simulink library "ammclib_bam"  (Simulink 9.3)
(part 5 of 21)

      |         add_block('built-in/Inport', [gcb, '/s16IntegGainShiftQ'], 'Position', pos, 'Orientation', orient, 'OutDataTypeStr', 'int16');
      | 
      |         pos = get_param(    [gcb, '/f32LowerLimitQ'], 'Position');
      |         orient = get_param( [gcb, '/f32LowerLimitQ'], 'Orientation');
      |         delete_block(       [gcb, '/f32LowerLimitQ']);
      |         add_block('built-in/Inport', [gcb, '/f32LowerLimitQ'], 'Position', pos, 'Orientation', orient, 'OutDataTypeStr', 'int32');
      | 
      |         pos = get_param(    [gcb, '/f32UpperLimitQ'], 'Position');
      |         orient = get_param( [gcb, '/f32UpperLimitQ'], 'Orientation');
      |         delete_block(       [gcb, '/f32UpperLimitQ']);
      |         add_block('built-in/Inport', [gcb, '/f32UpperLimitQ'], 'Position', pos, 'Orientation', orient, 'OutDataTypeStr', 'int32');
      | 
      |         pos = get_param(    [gcb, '/f32RampUp'], 'Position');
      |         orient = get_param( [gcb, '/f32RampUp'], 'Orientation');
      |         delete_block(       [gcb, '/f32RampUp']);
      |         add_block('built-in/Inport', [gcb, '/f32RampUp'], 'Position', pos, 'Orientation', orient, 'OutDataTypeStr', 'int32');
      | 
      |         pos = get_param(    [gcb, '/f32RampDown'], 'Position');
      |         orient = get_param( [gcb, '/f32RampDown'], 'Orientation');
      |         delete_block(       [gcb, '/f32RampDown']);
      |         add_block('built-in/Inport', [gcb, '/f32RampDown'], 'Position', pos, 'Orientation', orient, 'OutDataTypeStr', 'int32');
      | 
      |         pos = get_param(    [gcb, '/f32AccW'], 'Position');
      |         orient = get_param( [gcb, '/f32AccW'], 'Orientation');
      |         delete_block(       [gcb, '/f32AccW']);
      |         add_block('built-in/Inport', [gcb, '/f32AccW'], 'Position', pos, 'Orientation', orient, 'OutDataTypeStr', 'int32');
      | 
      |         pos = get_param(    [gcb, '/f32IntegPartK_1Q'], 'Position');
      |         orient = get_param( [gcb, '/f32IntegPartK_1Q'], 'Orientation');
      |         delete_block(       [gcb, '/f32IntegPartK_1Q']);
      |         add_block('built-in/Inport', [gcb, '/f32IntegPartK_1Q'], 'Position', pos, 'Orientation', orient, 'OutDataTypeStr', 'int32');
      | 
      |         pos = get_param(    [gcb, '/f32InK_1Q'], 'Position');
      |         orient = get_param( [gcb, '/f32InK_1Q'], 'Orientation');
      |         delete_block(       [gcb, '/f32InK_1Q']);
      |         add_block('built-in/Inport', [gcb, '/f32InK_1Q'], 'Position', pos, 'Orientation', orient, 'OutDataTypeStr', 'int32');
      | 
      |         pos = get_param(    [gcb, '/f32State'], 'Position');
      |         orient = get_param( [gcb, '/f32State'], 'Orientation');
      |         delete_block(       [gcb, '/f32State']);
      |         add_block('built-in/Inport', [gcb, '/f32State'], 'Position', pos, 'Orientation', orient, 'OutDataTypeStr', 'int32');
      | 
      | 
      |         pos = get_param(    [gcb '/f32AccW_Out'], 'Position');
      |         orient = get_param( [gcb '/f32AccW_Out'], 'Orientation');
      |         delete_block(       [gcb '/f32AccW_Out']);
      |         add_block('built-in/Outport', [gcb '/f32AccW_Out'], 'Position', pos, 'Orientation', orient);
      | 
      |         pos = get_param(    [gcb '/f32IntegPartK_1Q_Out'], 'Position');
      |         orient = get_param( [gcb '/f32IntegPartK_1Q_Out'], 'Orientation');
      |         delete_block(       [gcb '/f32IntegPartK_1Q_Out']);
      |         add_block('built-in/Outport', [gcb '/f32IntegPartK_1Q_Out'], 'Position', pos, 'Orientation', orient);
      | 
      |         pos = get_param(    [gcb '/f32InK_1Q_Out'], 'Position');
      |         orient = get_param( [gcb '/f32InK_1Q_Out'], 'Orientation');
      |         delete_block(       [gcb '/f32InK_1Q_Out']);
      |         add_block('built-in/Outport', [gcb '/f32InK_1Q_Out'], 'Position', pos, 'Orientation', orient);
      | 
      |         pos = get_param(    [gcb '/f32State_Out'], 'Position');
      |         orient = get_param( [gcb '/f32State_Out'], 'Orientation');
      |         delete_block(       [gcb '/f32State_Out']);
      |         add_block('built-in/Outport', [gcb '/f32State_Out'], 'Position', pos, 'Orientation', orient);
      | 
      | 
      |         if (showDebugOutputs == 2) && (strcmp(get_param([gcb '/f32WReqFilt'], 'BlockType'), 'Terminator'))
      |             pos = get_param(    [gcb '/f32WReqFilt'], 'Position');
      |             orient = get_param( [gcb '/f32WReqFilt'], 'Orientation');
      |             delete_block(       [gcb '/f32WReqFilt']);
      |             add_block('built-in/Outport', [gcb '/f32WReqFilt'], 'Position', pos, 'Orientation', orient);
      | 
      |             pos = get_param(    [gcb '/f32WErr'], 'Position');
      |             orient = get_param( [gcb '/f32WErr'], 'Orientation');
      |             delete_block(       [gcb '/f32WErr']);
      |             add_block('built-in/Outport', [gcb '/f32WErr'], 'Position', pos, 'Orientation', orient);
      | 
      |             pos = get_param(    [gcb '/f32WFbckFilt'], 'Position');
      |             orient = get_param( [gcb '/f32WFbckFilt'], 'Orientation');
      |             delete_block(       [gcb '/f32WFbckFilt']);
      |             add_block('built-in/Outport', [gcb '/f32WFbckFilt'], 'Position', pos, 'Orientation', orient);
      | 
      |         end
      | 
      |         set_param([gcb '/f32VelocityReq'], 'Port', '1');
      |         set_param([gcb '/f32VelocityFbck'], 'Port', '2');
      |         set_param([gcb '/f32FilterMAWOut_preset'], 'Port', '3');
      |         set_param([gcb '/f32ControllerPIpAWQOut_preset'], 'Port', '4');
      |         set_param([gcb '/f32RampOut_preset'], 'Port', '5');
      |         set_param([gcb '/u16NSamplesW'], 'Port', '6');
      |         set_param([gcb '/f32PropGainQ'], 'Port', '7');
      |         set_param([gcb '/f32IntegGainQ'], 'Port', '8');
      |         set_param([gcb '/s16PropGainShiftQ'], 'Port', '9');
      |         set_param([gcb '/s16IntegGainShiftQ'], 'Port', '10');
      |         set_param([gcb '/f32LowerLimitQ'], 'Port', '11');
      |         set_param([gcb '/f32UpperLimitQ'], 'Port', '12');
      |         set_param([gcb '/f32RampUp'], 'Port', '13');
      |         set_param([gcb '/f32RampDown'], 'Port', '14');
      |         set_param([gcb '/f32AccW'], 'Port', '15');
      |         set_param([gcb '/f32IntegPartK_1Q'], 'Port', '16');
      |         set_param([gcb '/f32InK_1Q'], 'Port', '17');
      |         set_param([gcb '/f32State'], 'Port', '18');
      | 
      |         if (showDebugOutputs == 2)
      |             set_param([gcb '/pIDQReq'], 'Port', '1');
      |             set_param([gcb '/u16LimitFlagQ'], 'Port', '2');
      |             set_param([gcb '/f32WReqFilt'], 'Port', '3');
      |             set_param([gcb '/f32WErr'], 'Port', '4');
      |             set_param([gcb '/f32WFbckFilt'], 'Port', '5');
      |             set_param([gcb '/f32AccW_Out'], 'Port', '6');
      |             set_param([gcb '/f32IntegPartK_1Q_Out'], 'Port', '7');
      |             set_param([gcb '/f32InK_1Q_Out'], 'Port', '8');
      |             set_param([gcb '/f32State_Out'], 'Port', '9');
      |         else
      |             set_param([gcb '/pIDQReq'], 'Port', '1');
      |             set_param([gcb '/u16LimitFlagQ'], 'Port', '2');
      |             set_param([gcb '/f32AccW_Out'], 'Port', '3');
      |             set_param([gcb '/f32IntegPartK_1Q_Out'], 'Port', '4');
      |             set_param([gcb '/f32InK_1Q_Out'], 'Port', '5');
      |             set_param([gcb '/f32State_Out'], 'Port', '6');
      |         end
      | 
      |         set_param(gcb,'MaskEnables',{'on','on','on','off','off','off','off','off','off','off','off','off'});
      | 
      |         if (posblk(4) - posblk(2)) < 475
      |           height = 475;
      |           set_param(gcb,'Position',[posblk(1), posblk(2), posblk(3), posblk(2)+height])
      |         end
      |     else
      |         if (showDebugOutputs == 2) && (strcmp(get_param([gcb '/f32WReqFilt'], 'BlockType'), 'Terminator'))
      |             % shown debugging outputs
      |             pos = get_param(    [gcb '/f32WReqFilt'], 'Position');
      |             orient = get_param( [gcb '/f32WReqFilt'], 'Orientation');
      |             delete_block(       [gcb '/f32WReqFilt']);
      |             add_block('built-in/Outport', [gcb '/f32WReqFilt'], 'Position', pos, 'Orientation', orient);
      | 
      |             pos = get_param(    [gcb '/f32WErr'], 'Position');
      |             orient = get_param( [gcb '/f32WErr'], 'Orientation');
      |             delete_block(       [gcb '/f32WErr']);
      |             add_block('built-in/Outport', [gcb '/f32WErr'], 'Position', pos, 'Orientation', orient);
      | 
      |             pos = get_param(    [gcb '/f32WFbckFilt'], 'Position');
      |             orient = get_param( [gcb '/f32WFbckFilt'], 'Orientation');
      |             delete_block(       [gcb '/f32WFbckFilt']);
      |             add_block('built-in/Outport', [gcb '/f32WFbckFilt'], 'Position', pos, 'Orientation', orient);
      | 
      |             set_param([gcb '/pIDQReq'], 'Port', '1');
      |             set_param([gcb '/u16LimitFlagQ'], 'Port', '2');
      |             set_param([gcb '/f32WReqFilt'], 'Port', '3');
      |             set_param([gcb '/f32WErr'], 'Port', '4');
      |             set_param([gcb '/f32WFbckFilt'], 'Port', '5');
      |             set_param([gcb '/f32AccW_Out'], 'Port', '6');
      |             set_param([gcb '/f32IntegPartK_1Q_Out'], 'Port', '7');
      |             set_param([gcb '/f32InK_1Q_Out'], 'Port', '8');
      |             set_param([gcb '/f32State_Out'], 'Port', '9');
      |         elseif (showDebugOutputs == 1) && (strcmp(get_param([gcb '/f32WReqFilt'], 'BlockType'), 'Outport'))
      |             % hidden debugging outputs
      |             pos = get_param(    [gcb '/f32WReqFilt'], 'Position');
      |             orient = get_param( [gcb '/f32WReqFilt'], 'Orientation');
      |             delete_block(       [gcb '/f32WReqFilt']);
      |             add_block('built-in/Terminator', [gcb '/f32WReqFilt'], 'Position', pos, 'Orientation', orient);
      | 
      |             pos = get_param(    [gcb '/f32WErr'], 'Position');
      |             orient = get_param( [gcb '/f32WErr'], 'Orientation');
      |             delete_block(       [gcb '/f32WErr']);
      |             add_block('built-in/Terminator', [gcb '/f32WErr'], 'Position', pos, 'Orientation', orient);
      | 
      |             pos = get_param(    [gcb '/f32WFbckFilt'], 'Position');
      |             orient = get_param( [gcb '/f32WFbckFilt'], 'Orientation');
      |             delete_block(       [gcb '/f32WFbckFilt']);
      |             add_block('built-in/Terminator', [gcb '/f32WFbckFilt'], 'Position', pos, 'Orientation', orient);
      | 
      |             set_param([gcb '/pIDQReq'], 'Port', '1');
      |             set_param([gcb '/u16LimitFlagQ'], 'Port', '2');
      |             set_param([gcb '/f32AccW_Out'], 'Port', '3');
      |             set_param([gcb '/f32IntegPartK_1Q_Out'], 'Port', '4');
      |             set_param([gcb '/f32InK_1Q_Out'], 'Port', '5');
      |             set_param([gcb '/f32State_Out'], 'Port', '6');
      |         end
      |     end
      | end
      settings: RTWSystemCode=Inline
      mask TypeOptions showStates: Hide (faster execution) | Show (allows debugging; connect feedback loops manually)
      mask Callback showStates:
      | maskStr = get_param(gcb,'showStates');
      | if strcmp(maskStr,'Hide (faster execution)'),
      |     set_param(gcb,'MaskEnables',{'on','on','off','on','on','on','on','on','on','on','on','on'});
      | else
      |     set_param(gcb,'MaskEnables',{'on','on','on','off','off','off','off','off','off','off','off','off'});
      | end
      mask TypeOptions resetStatesEnable: Pre-set according to the first set of inputs after reset | Clear to zero
      mask TypeOptions showDebugOutputs: Hide | Show
      mask Display:
      | color('black');
      | pos = get_param(gcb, 'Position');
      | width = pos(3) - pos(1);
      | height = pos(4) - pos(2);
      | tX=width/2;
      | tY=height - 25;
      | color('black');
      | text(tX,tY, 'AMCLIB_SpeedLoop_F32', 'horizontalAlignment', 'center');
      | if showStates == 2
      |   color('red');
      |   text(tX,tY - 20, ['debugging mode' char(13) char(10) '(limited performance)'], 'horizontalAlignment', 'center');
      | end
  AMCLIB_TrackObsrv_F32 : Subsystem  TreatAsAtomicUnit=on  mask(AMCLIB_TrackObsrv_F32){showStates=Hide (faster execution), resetStatesEnable=Pre-set according to the first set of inputs after reset, f32CC1sc=0, f32CC2sc=0, f32UpperLimit=0, f32LowerLimit=0, u16NShiftPI=0, f32C1=0, u16NShiftI=0}
      mask prompts: showStates "Show internal states"; resetStatesEnable "Internal state after reset"; f32CC1sc "f32CC1sc (GFLIB_ControllerPIrAW - CC1 coefficient)"; f32CC2sc "f32CC2sc (GFLIB_ControllerPIrAW - CC2 coefficient)"; f32UpperLimit "f32UpperLimit (GFLIB_ControllerPIrAW - upper Limit of the controller)"; f32LowerLimit "f32LowerLimit (GFLIB_ControllerPIrAW - lower Limit of the controller)"; u16NShiftPI "u16NShiftPI (GFLIB_ControllerPIrAW - scaling bitwise shift applied to the controller coefficients)"; f32C1 "f32C1 (GFLIB_IntegratorTR - integrator coefficient)"; u16NShiftI "u16NShiftI (GFLIB_IntegratorTR - scaling bitwise shift applied to the integrator coefficient)"
      mask help: Tracking observer in 32-bit fixed-point fractional implementation. This block supports re-initialization of the internal state during simulation. If the block is reset, the outputs of the PI controller and integrator will be aligned with the inputs f32VelocityOut_preset and f32PosOut_preset. Refer to the AMMCLIB User's Guide for further details.
      mask init:
      | if ~evalin('base','exist(''tS8'',''var'')')
      |   if (2 ~= exist('SWLIBS_Typedefs.mat','file'))
      |       error('File SWLIBS_Typedefs.mat is not on the Matlab path. Please add the AMMCLIB "bam" folder in the Matlab Search Path.');
      |   else
      |       evalin('base', 'load(''SWLIBS_Typedefs.mat'')');
      |   end
      | end
      | if showStates == 1
      |     % hidden state variables
      |     if strcmp(get_param([gcb '/f32CC1sc'], 'BlockType'), 'Inport')
      |         posblk = get_param(gcb, 'Position');
      | 
      |         pos = get_param(    [gcb, '/f32CC1sc'], 'Position');
      |         orient = get_param( [gcb, '/f32CC1sc'], 'Orientation');
      |         delete_block(       [gcb, '/f32CC1sc']);
      |         add_block('built-in/Ground', [gcb, '/f32CC1sc'], 'Position', pos, 'Orientation', orient);
      | 
      |         pos = get_param(    [gcb, '/f32CC2sc'], 'Position');
      |         orient = get_param( [gcb, '/f32CC2sc'], 'Orientation');
      |         delete_block(       [gcb, '/f32CC2sc']);
      |         add_block('built-in/Ground', [gcb, '/f32CC2sc'], 'Position', pos, 'Orientation', orient);
      | 
      |         pos = get_param(    [gcb, '/f32UpperLimit'], 'Position');
      |         orient = get_param( [gcb, '/f32UpperLimit'], 'Orientation');
      |         delete_block(       [gcb, '/f32UpperLimit']);
      |         add_block('built-in/Ground', [gcb, '/f32UpperLimit'], 'Position', pos, 'Orientation', orient);
      | 
      |         pos = get_param(    [gcb, '/f32LowerLimit'], 'Position');
      |         orient = get_param( [gcb, '/f32LowerLimit'], 'Orientation');
      |         delete_block(       [gcb, '/f32LowerLimit']);
      |         add_block('built-in/Ground', [gcb, '/f32LowerLimit'], 'Position', pos, 'Orientation', orient);
      | 
      |         pos = get_param(    [gcb, '/u16NShiftPI'], 'Position');
      |         orient = get_param( [gcb, '/u16NShiftPI'], 'Orientation');
      |         delete_block(       [gcb, '/u16NShiftPI']);
      |         add_block('built-in/Ground', [gcb, '/u16NShiftPI'], 'Position', pos, 'Orientation', orient);
      | 
      |         pos = get_param(    [gcb, '/f32C1'], 'Position');
      |         orient = get_param( [gcb, '/f32C1'], 'Orientation');
      |         delete_block(       [gcb, '/f32C1']);
      |         add_block('built-in/Ground', [gcb, '/f32C1'], 'Position', pos, 'Orientation', orient);
      | 
      |         pos = get_param(    [gcb, '/u16NShiftI'], 'Position');
      |         orient = get_param( [gcb, '/u16NShiftI'], 'Orientation');
      |         delete_block(       [gcb, '/u16NShiftI']);
      |         add_block('built-in/Ground', [gcb, '/u16NShiftI'], 'Position', pos, 'Orientation', orient);
      | 
      |         pos = get_param(    [gcb, '/f32Acc'], 'Position');
      |         orient = get_param( [gcb, '/f32Acc'], 'Orientation');
      |         delete_block(       [gcb, '/f32Acc']);
      |         add_block('built-in/Ground', [gcb, '/f32Acc'], 'Position', pos, 'Orientation', orient);
      | 
      |         pos = get_param(    [gcb, '/f32InErrK1'], 'Position');
      |         orient = get_param( [gcb, '/f32InErrK1'], 'Orientation');
      |         delete_block(       [gcb, '/f32InErrK1']);
      |         add_block('built-in/Ground', [gcb, '/f32InErrK1'], 'Position', pos, 'Orientation', orient);
      | 
      |         pos = get_param(    [gcb, '/f32State'], 'Position');
      |         orient = get_param( [gcb, '/f32State'], 'Orientation');
      |         delete_block(       [gcb, '/f32State']);
      |         add_block('built-in/Ground', [gcb, '/f32State'], 'Position', pos, 'Orientation', orient);
      | 
      |         pos = get_param(    [gcb, '/f32InK1'], 'Position');
      |         orient = get_param( [gcb, '/f32InK1'], 'Orientation');
      |         delete_block(       [gcb, '/f32InK1']);
      |         add_block('built-in/Ground', [gcb, '/f32InK1'], 'Position', pos, 'Orientation', orient);
      | 
      | 
      |         pos = get_param(    [gcb '/f32Acc_Out'], 'Position');
      |         orient = get_param( [gcb '/f32Acc_Out'], 'Orientation');
      |         delete_block(       [gcb '/f32Acc_Out']);
      |         add_block('built-in/Terminator', [gcb '/f32Acc_Out'], 'Position', pos, 'Orientation', orient);
      | 
      |         pos = get_param(    [gcb '/f32InErrK1_Out'], 'Position');
      |         orient = get_param( [gcb '/f32InErrK1_Out'], 'Orientation');
      |         delete_block(       [gcb '/f32InErrK1_Out']);
      |         add_block('built-in/Terminator', [gcb '/f32InErrK1_Out'], 'Position', pos, 'Orientation', orient);
      | 
      |         pos = get_param(    [gcb '/f32State_Out'], 'Position');
      |         orient = get_param( [gcb '/f32State_Out'], 'Orientation');
      |         delete_block(       [gcb '/f32State_Out']);
      |         add_block('built-in/Terminator', [gcb '/f32State_Out'], 'Position', pos, 'Orientation', orient);
      | 
      |         pos = get_param(    [gcb '/f32InK1_Out'], 'Position');
      |         orient = get_param( [gcb '/f32InK1_Out'], 'Orientation');
      |         delete_block(       [gcb '/f32InK1_Out']);
      |         add_block('built-in/Terminator', [gcb '/f32InK1_Out'], 'Position', pos, 'Orientation', orient);
      | 
      | 
      |         set_param([gcb '/f32PhaseErr'], 'Port', '1');
      |         set_param([gcb '/f32VelocityOut_preset'], 'Port', '2');
      |         set_param([gcb '/f32PosOut_preset'], 'Port', '3');
      | 
      |         set_param([gcb '/pPosEst'], 'Port', '1');
      |         set_param([gcb '/pVelocityEst'], 'Port', '2');
      | 
      |         set_param(gcb,'MaskEnables',{'on','on','on','on','on','on','on','on','on'});
      | 
      |         if (posblk(4) - posblk(2)) > 100
      |           height = 100;
      |           set_param(gcb,'Position',[posblk(1), posblk(2), posblk(3), posblk(2)+height])
      |         end
      |     end
      | else
      |     % shown state variables
      |     if strcmp(get_param([gcb '/f32CC1sc'], 'BlockType'), 'Ground')
      |         posblk = get_param(gcb, 'Position');
      | 
      |         pos = get_param(    [gcb, '/f32CC1sc'], 'Position');
      |         orient = get_param( [gcb, '/f32CC1sc'], 'Orientation');
      |         delete_block(       [gcb, '/f32CC1sc']);
      |         add_block('built-in/Inport', [gcb, '/f32CC1sc'], 'Position', pos, 'Orientation', orient, 'OutDataTypeStr', 'int32');
      | 
      |         pos = get_param(    [gcb, '/f32CC2sc'], 'Position');
      |         orient = get_param( [gcb, '/f32CC2sc'], 'Orientation');
      |         delete_block(       [gcb, '/f32CC2sc']);
      |         add_block('built-in/Inport', [gcb, '/f32CC2sc'], 'Position', pos, 'Orientation', orient, 'OutDataTypeStr', 'int32');
      | 
      |         pos = get_param(    [gcb, '/f32UpperLimit'], 'Position');
      |         orient = get_param( [gcb, '/f32UpperLimit'], 'Orientation');
      |         delete_block(       [gcb, '/f32UpperLimit']);
      |         add_block('built-in/Inport', [gcb, '/f32UpperLimit'], 'Position', pos, 'Orientation', orient, 'OutDataTypeStr', 'int32');
      | 
      |         pos = get_param(    [gcb, '/f32LowerLimit'], 'Position');
      |         orient = get_param( [gcb, '/f32LowerLimit'], 'Orientation');
      |         delete_block(       [gcb, '/f32LowerLimit']);
      |         add_block('built-in/Inport', [gcb, '/f32LowerLimit'], 'Position', pos, 'Orientation', orient, 'OutDataTypeStr', 'int32');
      | 
      |         pos = get_param(    [gcb, '/u16NShiftPI'], 'Position');
      |         orient = get_param( [gcb, '/u16NShiftPI'], 'Orientation');
      |         delete_block(       [gcb, '/u16NShiftPI']);
      |         add_block('built-in/Inport', [gcb, '/u16NShiftPI'], 'Position', pos, 'Orientation', orient, 'OutDataTypeStr', 'uint16');
      | 
      |         pos = get_param(    [gcb, '/f32C1'], 'Position');
      |         orient = get_param( [gcb, '/f32C1'], 'Orientation');
      |         delete_block(       [gcb, '/f32C1']);
      |         add_block('built-in/Inport', [gcb, '/f32C1'], 'Position', pos, 'Orientation', orient, 'OutDataTypeStr', 'int32');
      | 
      |         pos = get_param(    [gcb, '/u16NShiftI'], 'Position');
      |         orient = get_param( [gcb, '/u16NShiftI'], 'Orientation');
      |         delete_block(       [gcb, '/u16NShiftI']);
      |         add_block('built-in/Inport', [gcb, '/u16NShiftI'], 'Position', pos, 'Orientation', orient, 'OutDataTypeStr', 'uint16');
      | 
      |         pos = get_param(    [gcb, '/f32Acc'], 'Position');
      |         orient = get_param( [gcb, '/f32Acc'], 'Orientation');
      |         delete_block(       [gcb, '/f32Acc']);
      |         add_block('built-in/Inport', [gcb, '/f32Acc'], 'Position', pos, 'Orientation', orient, 'OutDataTypeStr', 'int32');
      | 
      |         pos = get_param(    [gcb, '/f32InErrK1'], 'Position');
      |         orient = get_param( [gcb, '/f32InErrK1'], 'Orientation');
      |         delete_block(       [gcb, '/f32InErrK1']);
      |         add_block('built-in/Inport', [gcb, '/f32InErrK1'], 'Position', pos, 'Orientation', orient, 'OutDataTypeStr', 'int32');
      | 
      |         pos = get_param(    [gcb, '/f32State'], 'Position');
      |         orient = get_param( [gcb, '/f32State'], 'Orientation');
      |         delete_block(       [gcb, '/f32State']);
      |         add_block('built-in/Inport', [gcb, '/f32State'], 'Position', pos, 'Orientation', orient, 'OutDataTypeStr', 'int32');
      | 
      |         pos = get_param(    [gcb, '/f32InK1'], 'Position');
      |         orient = get_param( [gcb, '/f32InK1'], 'Orientation');
      |         delete_block(       [gcb, '/f32InK1']);
      |         add_block('built-in/Inport', [gcb, '/f32InK1'], 'Position', pos, 'Orientation', orient, 'OutDataTypeStr', 'int32');
      | 
      | 
      |         pos = get_param(    [gcb '/f32Acc_Out'], 'Position');
      |         orient = get_param( [gcb '/f32Acc_Out'], 'Orientation');
      |         delete_block(       [gcb '/f32Acc_Out']);
      |         add_block('built-in/Outport', [gcb '/f32Acc_Out'], 'Position', pos, 'Orientation', orient);
      | 
      |         pos = get_param(    [gcb '/f32InErrK1_Out'], 'Position');
      |         orient = get_param( [gcb '/f32InErrK1_Out'], 'Orientation');
      |         delete_block(       [gcb '/f32InErrK1_Out']);
      |         add_block('built-in/Outport', [gcb '/f32InErrK1_Out'], 'Position', pos, 'Orientation', orient);
      | 
      |         pos = get_param(    [gcb '/f32State_Out'], 'Position');
      |         orient = get_param( [gcb '/f32State_Out'], 'Orientation');
      |         delete_block(       [gcb '/f32State_Out']);
      |         add_block('built-in/Outport', [gcb '/f32State_Out'], 'Position', pos, 'Orientation', orient);
      | 
      |         pos = get_param(    [gcb '/f32InK1_Out'], 'Position');
      |         orient = get_param( [gcb '/f32InK1_Out'], 'Orientation');
      |         delete_block(       [gcb '/f32InK1_Out']);
      |         add_block('built-in/Outport', [gcb '/f32InK1_Out'], 'Position', pos, 'Orientation', orient);
      | 
      | 
      |         set_param([gcb '/f32PhaseErr'], 'Port', '1');
      |         set_param([gcb '/f32VelocityOut_preset'], 'Port', '2');
      |         set_param([gcb '/f32PosOut_preset'], 'Port', '3');
      |         set_param([gcb '/f32CC1sc'], 'Port', '4');
      |         set_param([gcb '/f32CC2sc'], 'Port', '5');
      |         set_param([gcb '/f32UpperLimit'], 'Port', '6');
      |         set_param([gcb '/f32LowerLimit'], 'Port', '7');
      |         set_param([gcb '/u16NShiftPI'], 'Port', '8');
      |         set_param([gcb '/f32C1'], 'Port', '9');
      |         set_param([gcb '/u16NShiftI'], 'Port', '10');
      |         set_param([gcb '/f32Acc'], 'Port', '11');
      |         set_param([gcb '/f32InErrK1'], 'Port', '12');
      |         set_param([gcb '/f32State'], 'Port', '13');
      |         set_param([gcb '/f32InK1'], 'Port', '14');
      | 
      |         set_param([gcb '/pPosEst'], 'Port', '1');
      |         set_param([gcb '/pVelocityEst'], 'Port', '2');
      |         set_param([gcb '/f32Acc_Out'], 'Port', '3');
      |         set_param([gcb '/f32InErrK1_Out'], 'Port', '4');
      |         set_param([gcb '/f32State_Out'], 'Port', '5');
      |         set_param([gcb '/f32InK1_Out'], 'Port', '6');
      | 
      |         set_param(gcb,'MaskEnables',{'on','on','off','off','off','off','off','off','off'});
      | 
      |         if (posblk(4) - posblk(2)) < 375
      |           height = 375;
      |           set_param(gcb,'Position',[posblk(1), posblk(2), posblk(3), posblk(2)+height])
      |         end
      |     end
      | end
      settings: RTWSystemCode=Inline
      mask TypeOptions showStates: Hide (faster execution) | Show (allows debugging; connect feedback loops manually)
      mask Callback showStates:
      | maskStr = get_param(gcb,'showStates');
      | if strcmp(maskStr,'Hide (faster execution)'),
      |     set_param(gcb,'MaskEnables',{'on','on','on','on','on','on','on','on','on'});
      | else
      |     set_param(gcb,'MaskEnables',{'on','on','off','off','off','off','off','off','off'});
      | end
      mask TypeOptions resetStatesEnable: Pre-set according to the first set of inputs after reset | Clear to zero
      mask Display:
      | color('black');
      | pos = get_param(gcb, 'Position');
      | width = pos(3) - pos(1);
      | height = pos(4) - pos(2);
      | tX=width/2;
      | tY=height - 25;
      | color('black');
      | text(tX,tY, 'AMCLIB_TrackObsrv_F32', 'horizontalAlignment', 'center');
      | if showStates == 2
      |   color('red');
      |   text(tX,tY - 20, ['debugging mode' char(13) char(10) '(limited performance)'], 'horizontalAlignment', 'center');
      | end
  AMCLIB_Windmilling_F32 : Subsystem  TreatAsAtomicUnit=on  mask(AMCLIB_Windmilling_F32){showStates=Hide (faster execution), f32ADCMaxError=0, f32CC1sc=0, f32CC2sc=0, f32UpperLimit=0, f32LowerLimit=0, u16NShiftPI=0, f32C1=0, u16NShiftI=0}
      mask prompts: showStates "Show internal states"; f32ADCMaxError "f32ADCMaxError (Maximum differential offset error between any two phases of the 3-phase voltage-sensing A/D converters.)"; f32CC1sc "f32CC1sc (GFLIB_ControllerPIrAW - CC1 coefficient)"; f32CC2sc "f32CC2sc (GFLIB_ControllerPIrAW - CC2 coefficient)"; f32UpperLimit "f32UpperLimit (GFLIB_ControllerPIrAW - upper Limit of the controller)"; f32LowerLimit "f32LowerLimit (GFLIB_ControllerPIrAW - lower Limit of the controller)"; u16NShiftPI "u16NShiftPI (GFLIB_ControllerPIrAW - scaling bitwise shift applied to the controller coefficients)"; f32C1 "f32C1 (GFLIB_IntegratorTR - integrator coefficient)"; u16NShiftI "u16NShiftI (GFLIB_IntegratorTR - scaling bitwise shift applied to the integrator coefficient)"
      mask help: PMSM Windmilling in 32-bit fixed-point fractional implementation. This function detects spontaneous rotation of an unpowered 3-phase PMSM by measuring the generated back electromotive force. Output u32Lock represents the return value of the C function (0 = undecided, 1 = spinning, 2 = stopped). Transition from 0 to 1 on the u32Lock output can be taken as a reset signal for the following AMCLIB_TrackObsrv_F32 block to synchronize the sensorless FOC loop with a freewheeling motor. Refer to the AMMCLIB User's Guide for further details.
      mask init:
      | if ~evalin('base','exist(''tS8'',''var'')')
      |   if (2 ~= exist('SWLIBS_Typedefs.mat','file'))
      |       error('File SWLIBS_Typedefs.mat is not on the Matlab path. Please add the AMMCLIB "bam" folder in the Matlab Search Path.');
      |   else
      |       evalin('base', 'load(''SWLIBS_Typedefs.mat'')');
      |   end
      | end
      | if showStates == 1
      |     % hidden state variables
      |     if strcmp(get_param([gcb '/f32ADCMaxError'], 'BlockType'), 'Inport')
      |         posblk = get_param(gcb, 'Position');
      | 
      |         pos = get_param(    [gcb, '/f32ADCMaxError'], 'Position');
      |         orient = get_param( [gcb, '/f32ADCMaxError'], 'Orientation');
      |         delete_block(       [gcb, '/f32ADCMaxError']);
      |         add_block('built-in/Ground', [gcb, '/f32ADCMaxError'], 'Position', pos, 'Orientation', orient);
      | 
      |         pos = get_param(    [gcb, '/f32CC1sc'], 'Position');
      |         orient = get_param( [gcb, '/f32CC1sc'], 'Orientation');
      |         delete_block(       [gcb, '/f32CC1sc']);
      |         add_block('built-in/Ground', [gcb, '/f32CC1sc'], 'Position', pos, 'Orientation', orient);
      | 
      |         pos = get_param(    [gcb, '/f32CC2sc'], 'Position');
      |         orient = get_param( [gcb, '/f32CC2sc'], 'Orientation');
      |         delete_block(       [gcb, '/f32CC2sc']);
      |         add_block('built-in/Ground', [gcb, '/f32CC2sc'], 'Position', pos, 'Orientation', orient);
      | 
      |         pos = get_param(    [gcb, '/f32UpperLimit'], 'Position');
      |         orient = get_param( [gcb, '/f32UpperLimit'], 'Orientation');
      |         delete_block(       [gcb, '/f32UpperLimit']);
      |         add_block('built-in/Ground', [gcb, '/f32UpperLimit'], 'Position', pos, 'Orientation', orient);
      | 
      |         pos = get_param(    [gcb, '/f32LowerLimit'], 'Position');
      |         orient = get_param( [gcb, '/f32LowerLimit'], 'Orientation');
      |         delete_block(       [gcb, '/f32LowerLimit']);
      |         add_block('built-in/Ground', [gcb, '/f32LowerLimit'], 'Position', pos, 'Orientation', orient);
      | 
      |         pos = get_param(    [gcb, '/u16NShiftPI'], 'Position');
      |         orient = get_param( [gcb, '/u16NShiftPI'], 'Orientation');
      |         delete_block(       [gcb, '/u16NShiftPI']);
      |         add_block('built-in/Ground', [gcb, '/u16NShiftPI'], 'Position', pos, 'Orientation', orient);
      | 
      |         pos = get_param(    [gcb, '/f32C1'], 'Position');
      |         orient = get_param( [gcb, '/f32C1'], 'Orientation');
      |         delete_block(       [gcb, '/f32C1']);
      |         add_block('built-in/Ground', [gcb, '/f32C1'], 'Position', pos, 'Orientation', orient);
      | 
      |         pos = get_param(    [gcb, '/u16NShiftI'], 'Position');
      |         orient = get_param( [gcb, '/u16NShiftI'], 'Orientation');
      |         delete_block(       [gcb, '/u16NShiftI']);
      |         add_block('built-in/Ground', [gcb, '/u16NShiftI'], 'Position', pos, 'Orientation', orient);
      | 
      |         pos = get_param(    [gcb, '/f32AccPI'], 'Position');
      |         orient = get_param( [gcb, '/f32AccPI'], 'Orientation');
      |         delete_block(       [gcb, '/f32AccPI']);
      |         add_block('built-in/Ground', [gcb, '/f32AccPI'], 'Position', pos, 'Orientation', orient);
      | 
      |         pos = get_param(    [gcb, '/f32InErrK1'], 'Position');
      |         orient = get_param( [gcb, '/f32InErrK1'], 'Orientation');
      |         delete_block(       [gcb, '/f32InErrK1']);
      |         add_block('built-in/Ground', [gcb, '/f32InErrK1'], 'Position', pos, 'Orientation', orient);
      | 
      |         pos = get_param(    [gcb, '/f32State'], 'Position');
      |         orient = get_param( [gcb, '/f32State'], 'Orientation');
      |         delete_block(       [gcb, '/f32State']);
      |         add_block('built-in/Ground', [gcb, '/f32State'], 'Position', pos, 'Orientation', orient);
      | 
      |         pos = get_param(    [gcb, '/f32InK1'], 'Position');
      |         orient = get_param( [gcb, '/f32InK1'], 'Orientation');
      |         delete_block(       [gcb, '/f32InK1']);
      |         add_block('built-in/Ground', [gcb, '/f32InK1'], 'Position', pos, 'Orientation', orient);
      | 
      | 
      |         pos = get_param(    [gcb '/f32AccPI_Out'], 'Position');
      |         orient = get_param( [gcb '/f32AccPI_Out'], 'Orientation');
      |         delete_block(       [gcb '/f32AccPI_Out']);
      |         add_block('built-in/Terminator', [gcb '/f32AccPI_Out'], 'Position', pos, 'Orientation', orient);
      | 
      |         pos = get_param(    [gcb '/f32InErrK1_Out'], 'Position');
      |         orient = get_param( [gcb '/f32InErrK1_Out'], 'Orientation');
      |         delete_block(       [gcb '/f32InErrK1_Out']);
      |         add_block('built-in/Terminator', [gcb '/f32InErrK1_Out'], 'Position', pos, 'Orientation', orient);
      | 
      |         pos = get_param(    [gcb '/f32State_Out'], 'Position');
      |         orient = get_param( [gcb '/f32State_Out'], 'Orientation');
      |         delete_block(       [gcb '/f32State_Out']);
      |         add_block('built-in/Terminator', [gcb '/f32State_Out'], 'Position', pos, 'Orientation', orient);
      | 
      |         pos = get_param(    [gcb '/f32InK1_Out'], 'Position');
      |         orient = get_param( [gcb '/f32InK1_Out'], 'Orientation');
      |         delete_block(       [gcb '/f32InK1_Out']);
      |         add_block('built-in/Terminator', [gcb '/f32InK1_Out'], 'Position', pos, 'Orientation', orient);
      | 
      | 
      |         set_param([gcb '/pUabcIn'], 'Port', '1');
      | 
      |         set_param([gcb '/u32Lock'], 'Port', '1');
      |         set_param([gcb '/pPosEst'], 'Port', '2');
      |         set_param([gcb '/pVelocityEst'], 'Port', '3');
      | 
      |         set_param(gcb,'MaskEnables',{'on','on','on','on','on','on','on','on','on'});
      | 
      |         if (posblk(4) - posblk(2)) > 100
      |           height = 100;
      |           set_param(gcb,'Position',[posblk(1), posblk(2), posblk(3), posblk(2)+height])
      |         end
      |     end
      | else
      |     % shown state variables
      |     if strcmp(get_param([gcb '/f32ADCMaxError'], 'BlockType'), 'Ground')
      |         posblk = get_param(gcb, 'Position');
      | 
      |         pos = get_param(    [gcb, '/f32ADCMaxError'], 'Position');
      |         orient = get_param( [gcb, '/f32ADCMaxError'], 'Orientation');
      |         delete_block(       [gcb, '/f32ADCMaxError']);
      |         add_block('built-in/Inport', [gcb, '/f32ADCMaxError'], 'Position', pos, 'Orientation', orient, 'OutDataTypeStr', 'int32');
      | 
      |         pos = get_param(    [gcb, '/f32CC1sc'], 'Position');
      |         orient = get_param( [gcb, '/f32CC1sc'], 'Orientation');
      |         delete_block(       [gcb, '/f32CC1sc']);
      |         add_block('built-in/Inport', [gcb, '/f32CC1sc'], 'Position', pos, 'Orientation', orient, 'OutDataTypeStr', 'int32');
      | 
      |         pos = get_param(    [gcb, '/f32CC2sc'], 'Position');
      |         orient = get_param( [gcb, '/f32CC2sc'], 'Orientation');
      |         delete_block(       [gcb, '/f32CC2sc']);
      |         add_block('built-in/Inport', [gcb, '/f32CC2sc'], 'Position', pos, 'Orientation', orient, 'OutDataTypeStr', 'int32');
      | 
      |         pos = get_param(    [gcb, '/f32UpperLimit'], 'Position');
      |         orient = get_param( [gcb, '/f32UpperLimit'], 'Orientation');
      |         delete_block(       [gcb, '/f32UpperLimit']);
      |         add_block('built-in/Inport', [gcb, '/f32UpperLimit'], 'Position', pos, 'Orientation', orient, 'OutDataTypeStr', 'int32');
      | 
      |         pos = get_param(    [gcb, '/f32LowerLimit'], 'Position');
      |         orient = get_param( [gcb, '/f32LowerLimit'], 'Orientation');
      |         delete_block(       [gcb, '/f32LowerLimit']);
      |         add_block('built-in/Inport', [gcb, '/f32LowerLimit'], 'Position', pos, 'Orientation', orient, 'OutDataTypeStr', 'int32');
      | 
      |         pos = get_param(    [gcb, '/u16NShiftPI'], 'Position');
      |         orient = get_param( [gcb, '/u16NShiftPI'], 'Orientation');
      |         delete_block(       [gcb, '/u16NShiftPI']);
      |         add_block('built-in/Inport', [gcb, '/u16NShiftPI'], 'Position', pos, 'Orientation', orient, 'OutDataTypeStr', 'uint16');
      | 
      |         pos = get_param(    [gcb, '/f32C1'], 'Position');
      |         orient = get_param( [gcb, '/f32C1'], 'Orientation');
      |         delete_block(       [gcb, '/f32C1']);
      |         add_block('built-in/Inport', [gcb, '/f32C1'], 'Position', pos, 'Orientation', orient, 'OutDataTypeStr', 'int32');
      | 
      |         pos = get_param(    [gcb, '/u16NShiftI'], 'Position');
      |         orient = get_param( [gcb, '/u16NShiftI'], 'Orientation');
      |         delete_block(       [gcb, '/u16NShiftI']);
      |         add_block('built-in/Inport', [gcb, '/u16NShiftI'], 'Position', pos, 'Orientation', orient, 'OutDataTypeStr', 'uint16');
      | 
      |         pos = get_param(    [gcb, '/f32AccPI'], 'Position');
      |         orient = get_param( [gcb, '/f32AccPI'], 'Orientation');
      |         delete_block(       [gcb, '/f32AccPI']);
      |         add_block('built-in/Inport', [gcb, '/f32AccPI'], 'Position', pos, 'Orientation', orient, 'OutDataTypeStr', 'int32');
      | 
      |         pos = get_param(    [gcb, '/f32InErrK1'], 'Position');
      |         orient = get_param( [gcb, '/f32InErrK1'], 'Orientation');
      |         delete_block(       [gcb, '/f32InErrK1']);
      |         add_block('built-in/Inport', [gcb, '/f32InErrK1'], 'Position', pos, 'Orientation', orient, 'OutDataTypeStr', 'int32');
      | 
      |         pos = get_param(    [gcb, '/f32State'], 'Position');
      |         orient = get_param( [gcb, '/f32State'], 'Orientation');
      |         delete_block(       [gcb, '/f32State']);
      |         add_block('built-in/Inport', [gcb, '/f32State'], 'Position', pos, 'Orientation', orient, 'OutDataTypeStr', 'int32');
      | 
      |         pos = get_param(    [gcb, '/f32InK1'], 'Position');
      |         orient = get_param( [gcb, '/f32InK1'], 'Orientation');
      |         delete_block(       [gcb, '/f32InK1']);
      |         add_block('built-in/Inport', [gcb, '/f32InK1'], 'Position', pos, 'Orientation', orient, 'OutDataTypeStr', 'int32');
      | 
      | 
      |         pos = get_param(    [gcb '/f32AccPI_Out'], 'Position');
      |         orient = get_param( [gcb '/f32AccPI_Out'], 'Orientation');
      |         delete_block(       [gcb '/f32AccPI_Out']);
      |         add_block('built-in/Outport', [gcb '/f32AccPI_Out'], 'Position', pos, 'Orientation', orient);
      | 
      |         pos = get_param(    [gcb '/f32InErrK1_Out'], 'Position');
      |         orient = get_param( [gcb '/f32InErrK1_Out'], 'Orientation');
      |         delete_block(       [gcb '/f32InErrK1_Out']);
      |         add_block('built-in/Outport', [gcb '/f32InErrK1_Out'], 'Position', pos, 'Orientation', orient);
      | 
      |         pos = get_param(    [gcb '/f32State_Out'], 'Position');
      |         orient = get_param( [gcb '/f32State_Out'], 'Orientation');
      |         delete_block(       [gcb '/f32State_Out']);
      |         add_block('built-in/Outport', [gcb '/f32State_Out'], 'Position', pos, 'Orientation', orient);
      | 
      |         pos = get_param(    [gcb '/f32InK1_Out'], 'Position');
      |         orient = get_param( [gcb '/f32InK1_Out'], 'Orientation');
      |         delete_block(       [gcb '/f32InK1_Out']);
      |         add_block('built-in/Outport', [gcb '/f32InK1_Out'], 'Position', pos, 'Orientation', orient);
      | 
      | 
      |         set_param([gcb '/pUabcIn'], 'Port', '1');
      |         set_param([gcb '/f32ADCMaxError'], 'Port', '2');
      |         set_param([gcb '/f32CC1sc'], 'Port', '3');
      |         set_param([gcb '/f32CC2sc'], 'Port', '4');
      |         set_param([gcb '/f32UpperLimit'], 'Port', '5');
      |         set_param([gcb '/f32LowerLimit'], 'Port', '6');
      |         set_param([gcb '/u16NShiftPI'], 'Port', '7');
      |         set_param([gcb '/f32C1'], 'Port', '8');
      |         set_param([gcb '/u16NShiftI'], 'Port', '9');
      |         set_param([gcb '/f32AccPI'], 'Port', '10');
      |         set_param([gcb '/f32InErrK1'], 'Port', '11');
      |         set_param([gcb '/f32State'], 'Port', '12');
      |         set_param([gcb '/f32InK1'], 'Port', '13');
      | 
      |         set_param([gcb '/u32Lock'], 'Port', '1');
      |         set_param([gcb '/pPosEst'], 'Port', '2');
      |         set_param([gcb '/pVelocityEst'], 'Port', '3');
      |         set_param([gcb '/f32AccPI_Out'], 'Port', '4');
      |         set_param([gcb '/f32InErrK1_Out'], 'Port', '5');
      |         set_param([gcb '/f32State_Out'], 'Port', '6');
      |         set_param([gcb '/f32InK1_Out'], 'Port', '7');
      | 
      |         set_param(gcb,'MaskEnables',{'on','off','off','off','off','off','off','off','off'});
      | 
      |         if (posblk(4) - posblk(2)) < 350
      |           height = 350;
      |           set_param(gcb,'Position',[posblk(1), posblk(2), posblk(3), posblk(2)+height])
      |         end
      |     end
      | end
      settings: RTWSystemCode=Inline
      mask TypeOptions showStates: Hide (faster execution) | Show (allows debugging; connect feedback loops manually)
      mask Callback showStates:
      | maskStr = get_param(gcb,'showStates');
      | if strcmp(maskStr,'Hide (faster execution)'),
      |     set_param(gcb,'MaskEnables',{'on','on','on','on','on','on','on','on','on'});
      | else
      |     set_param(gcb,'MaskEnables',{'on','off','off','off','off','off','off','off','off'});
      | end
      mask Display:
      | color('black');
      | pos = get_param(gcb, 'Position');
      | width = pos(3) - pos(1);
      | height = pos(4) - pos(2);
      | tX=width/2;
      | tY=height - 8;
      | color('black');
      | text(tX,tY, 'AMCLIB_Windmilling_F32', 'horizontalAlignment', 'center');
      | if showStates == 2
      |   color('red');
      |   text(tX,tY - 20, ['debugging mode' char(13) char(10) '(limited performance)'], 'horizontalAlignment', 'center');
      | end
